simulink model "model_3dof_lateral_carsim"  (R2022a)
settings: Solver=ode5  StartTime=0.0  StopTime=1200  FixedStep=para_sim_step  MaxStep=1e-3  RelTol=1e-3
model workspace (MAT data in the model file):
  SCD_FRESTIMATE_Operating_Point = opcond.OperatingPoint
  SCD_FRESTIMATE_Operating_Point.Model_ = 'model_1dof_longitudinal'
  SCD_FRESTIMATE_Operating_Point.States_(1) = opcond.StatePoint
  SCD_FRESTIMATE_Operating_Point.States_(1).Nx_ = 41
  SCD_FRESTIMATE_Operating_Point.States_(1).Block_ = 'model_1dof_longitudinal/Excitation System/Int Operator'
  SCD_FRESTIMATE_Operating_Point.States_(1).StateName_ = 'v'
  SCD_FRESTIMATE_Operating_Point.States_(1).x_ = [2.02683501926e-10; 1.37568821264e-19; 7.14890844399e-22; 1.12455204277e-20; -7.0630005675e-20; -6.95938068614e-20; 2.72721447959e-21; -3.93535312325e-20; -1.14815977745e-19; 3.30570889294e-20; 3.78600196645e-20; 7.21851569254e-20; -1.77555585105e-19; -2.35291525241e-20; 4.41713994739e-20; -2.05900764101e-21; -1.58367864176e-20; 6.35039836383e-20; -1.30347120926e-20; 1.28680290784e-21; 5.17371795703e-20; 6.49899736287e-20; -4.65181773693e-21; 5.74556218522e-21; -3.90326541642e-20; -4.95314223748e-20; -4.80167923753e-19; 9.22449192438e-20; -2.20085792962e-21; -4.30092800651e-20; -3.42774380714e-20; -1.20947897418e-20; -3.0642370533e-20; -6.43164282462e-20; -2.97515387843e-19; -1.68698506591e-20; 2.312266433e-19; -7.84373380068e-21; 1.67577252929e-20; 2.59801809162e-21; -7.43993193604e-23]
  SCD_FRESTIMATE_Operating_Point.States_(2) = opcond.StatePoint
  SCD_FRESTIMATE_Operating_Point.States_(2).Nx_ = 1
  SCD_FRESTIMATE_Operating_Point.States_(2).Block_ = 'model_1dof_longitudinal/Vehicle Body 1DOF Longitudinal/Vehicle Body 1 DOF/Bus Creation/Body Frame/Longitudinal 1DOF/Integrator3'
  SCD_FRESTIMATE_Operating_Point.States_(2).x_ = 7.28555022085e-16
  SCD_FRESTIMATE_Operating_Point.States_(3) = opcond.StatePoint
  SCD_FRESTIMATE_Operating_Point.States_(3).Nx_ = 1
  SCD_FRESTIMATE_Operating_Point.States_(3).Block_ = 'model_1dof_longitudinal/Vehicle Body 1DOF Longitudinal/Vehicle Body 1 DOF/Integrator1'
  SCD_FRESTIMATE_Operating_Point.States_(3).x_ = -8.63730588445e-16
  SCD_FRESTIMATE_Operating_Point.States_(4) = opcond.StatePoint
  SCD_FRESTIMATE_Operating_Point.States_(4).Nx_ = 1
  SCD_FRESTIMATE_Operating_Point.States_(4).Block_ = 'model_1dof_longitudinal/Vehicle Body 1DOF Longitudinal/Vehicle Body 1 DOF/Vehicle/Integrator'
  SCD_FRESTIMATE_Operating_Point.States_(4).x_ = 1.82750662194e-20
values from neighbouring files (symbols this model uses):
  para_mats = paraStruct.Sv    [main_lateral.m]    (also in main_steering_lateral.m)
  para_sim_matu = paraStruct.SimUv    [main_lateral.m]    (also in main_steering_lateral.m)
  para_sim_step = 5e-4/2    (= 0.00025)    [main_lateral.m]    (also in main_steering_lateral.m = 0.005)
  para_vinit = paraStruct.VInit    [main_lateral.m]    (also in main_steering_lateral.m)
  sim_iun = Simulink.Parameter(1)    [main_lateral.m]    (also in main_steering_lateral.m)
  sim_usnr = zeros(para_sim_usize, 1)    [main_lateral.m]    (also in main_steering_lateral.m)
  ut_pwr = genPower(sim_ut, para_sim_usize)    [main_lateral.m]    (also in main_steering_lateral.m)
libraries: Solver_SF x1, simulink x1
settings Model: SimulationMode=accelerator  Creator=无垠穹宇  LastModifiedBy=无垠穹宇
settings DataIOCC: SaveOutput=off  SignalLogging=off  DSMLogging=off  SignalLoggingName=yt
settings OptimizationCC: SimCompilerOptimization=on
settings DebuggingCC: AlgebraicLoopMsg=none
settings SFSimCC: SimHardwareAcceleration=native
settings RTWCC: DLArmComputeVersion=19.05

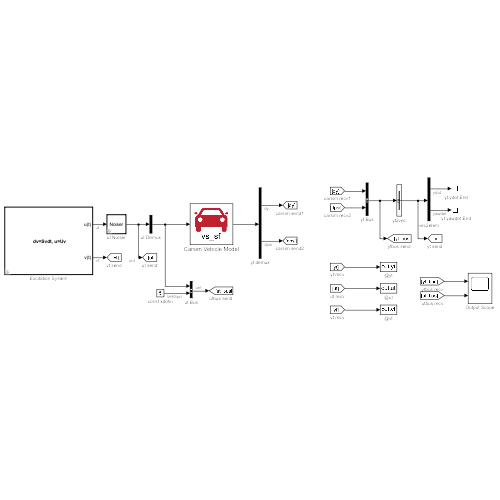
[thumbnail: Simulink's stored preview of the top-level diagram]
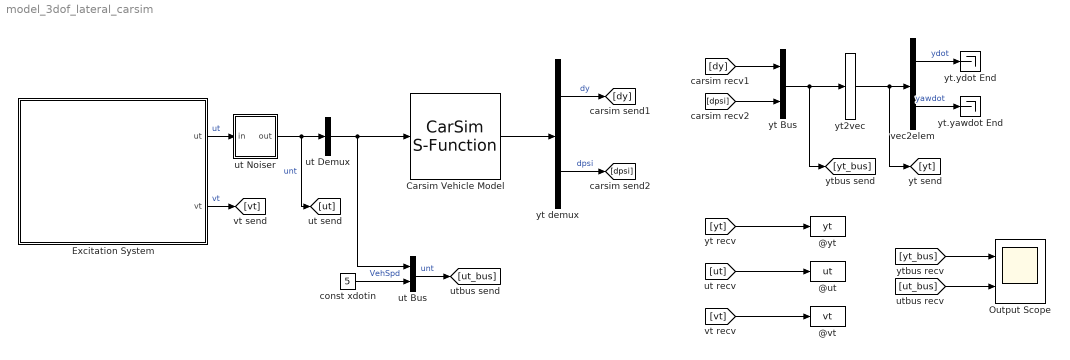
== system model_3dof_lateral_carsim ==
  @ut : ToWorkspace  VariableName=ut  SaveFormat=Timeseries  SampleTime=para_sim_step
      settings: Decimation=para_resamples
  @vt : ToWorkspace  VariableName=vt  SaveFormat=Timeseries  SampleTime=para_sim_step
      settings: Decimation=para_resamples
  @yt : ToWorkspace  VariableName=yt  SaveFormat=Timeseries  SampleTime=para_sim_step
      settings: Decimation=para_resamples
  Carsim Vehicle Model : Solver_SF/CarSim S-Function  Priority=1  SIMFILE=simfile.sim  Run_RTs=off  vs_state_ind=Run  StopMode_ind=Vehicle Model
  Excitation System : Subsystem  TreatAsAtomicUnit=on  mask(State Space with State Vector Output){S=para_mats, U=para_sim_matu, v0=para_vinit}
      mask prompts: S "Matrix S"; U "Matrix U"; v0 "v(0)"
      mask help: 带状态输出的状态空间模型(无控制输入)
      mask DialogControl ParameterGroupVar Prompt: 参数
      mask Display:
      | disp('\bf dv=Svdt, u=Uv', 'texmode', 'on');
      | port_label('output', 1, 'u(t)');
      | port_label('output', 2, 'v(t)');
  Output Scope : Scope  NumInputPorts=2
  const xdotin : Constant  Value=5  VectorParams1D=off  OutDataTypeStr=double
  ut Bus : BusCreator  Inputs=2
  ut Demux : Demux  Outputs=1
  ut Noiser : Subsystem  TreatAsAtomicUnit=on  mask(Vectorized AWGN){pwr=ut_pwr, snr=sim_usnr, tmin=20*para_sim_step, judge_para=sim_iun}
      mask prompts: pwr "信号功率向量 (W)"; snr "信噪比向量   (dB)"; tmin "最小动态时间 (s)"; judge_para "噪声启用判断"
      mask help: 给定信号功率和信噪比, 添加高斯白噪声到信号中
      mask DialogControl ParameterGroupVar Prompt: 参数
      mask Display: disp('Noiser');
  vec2elem : Demux  Outputs=2
  yt Bus : BusCreator  Inputs=2
  yt demux : Demux  Outputs=2
  yt.yawdot End : Terminator
  yt.ydot End : Terminator
  yt2vec : BusToVector
  wires:
  Excitation System/1(ut) -> ut Noiser/1(in)  "ut"
  ut Noiser/1(out) -> ut Demux/1, [ut]  "unt"
  Excitation System/2(vt) -> [vt]  "vt"
  [vt] -> @vt/1
  yt Bus/1 -> yt2vec/1, [yt_bus]
  [ut_bus] -> Output Scope/2
  [ut] -> @ut/1
  [yt_bus] -> Output Scope/1
  [yt] -> @yt/1
  yt2vec/1 -> vec2elem/1, [yt]
  Carsim Vehicle Model/1 -> yt demux/1
  yt demux/1 -> [dy]  "dy"
  yt demux/2 -> [dpsi]  "dpsi"
  const xdotin/1 -> ut Bus/2  "VehSpd"
  ut Bus/1 -> [ut_bus]  "unt"
  ut Demux/1 -> ut Bus/1, Carsim Vehicle Model/1
  [dy] -> yt Bus/1
  [dpsi] -> yt Bus/2
  vec2elem/1 -> yt.ydot End/1  "ydot"
  vec2elem/2 -> yt.yawdot End/1  "yawdot"

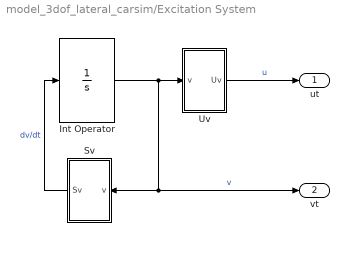
== system model_3dof_lateral_carsim/Excitation System ==
  Int Operator : Integrator  InitialCondition=v0  ContinuousStateAttributes='v'
  Sv : Subsystem
      mask Display: disp('Sv');
  Uv : Subsystem
      mask Display: disp('Uv');
  ut : Outport  OutDataTypeStr=double
  vt : Outport  Port=2  OutDataTypeStr=double
  wires:
  Uv/1(Uv) -> ut/1  "u"
  Int Operator/1 -> Uv/1(v), vt/1, Sv/1(v)  "v"
  Sv/1(Sv) -> Int Operator/1  "dv/dt"

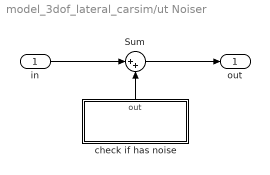
== system model_3dof_lateral_carsim/ut Noiser ==
  in : Inport  OutDataTypeStr=double
  Sum : Sum  Inputs=|++  AccumDataTypeStr=double  OutDataTypeStr=double
  check if has noise : Subsystem  Variant=on
      mask Display: disp('Variant: awgn/zeros');
  out : Outport  OutDataTypeStr=double
  wires:
  in/1 -> Sum/1
  Sum/1 -> out/1
  check if has noise/1(out) -> Sum/2

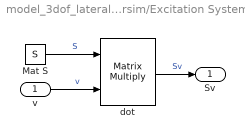
== system model_3dof_lateral_carsim/Excitation System/Sv ==
  v : Inport  OutDataTypeStr=double
  Mat S : Constant  Value=S  VectorParams1D=off  OutDataTypeStr=double
  dot : Product  Multiplication=Matrix(*)  InputSameDT=on  OutDataTypeStr=double
  Sv : Outport  OutDataTypeStr=double
  wires:
  dot/1 -> Sv/1  "Sv"
  v/1 -> dot/2  "v"
  Mat S/1 -> dot/1  "S"

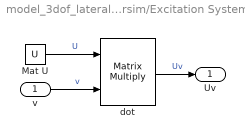
== system model_3dof_lateral_carsim/Excitation System/Uv ==
  v : Inport  OutDataTypeStr=double
  Mat U : Constant  Value=U  VectorParams1D=off  OutDataTypeStr=double
  dot : Product  Multiplication=Matrix(*)  InputSameDT=on  OutDataTypeStr=double
  Uv : Outport  OutDataTypeStr=double
  wires:
  dot/1 -> Uv/1  "Uv"
  Mat U/1 -> dot/1  "U"
  v/1 -> dot/2  "v"

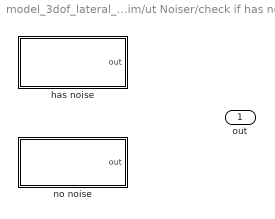
== system model_3dof_lateral_carsim/ut Noiser/check if has noise ==
  has noise : Subsystem  TreatAsAtomicUnit=on  VariantControl=judge_para == 0
  no noise : Subsystem  TreatAsAtomicUnit=on  VariantControl=judge_para ~= 0
  out : Outport  OutDataTypeStr=double

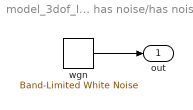
== system model_3dof_lateral_carsim/ut Noiser/check if has noise/has noise ==
  wgn : simulink/Sources/Band-Limited White Noise  Cov=pwr./(10.^(snr./10)).*(2*pi*tmin/100)  Ts=(1/20)*tmin  seed=[23341]
  out : Outport  OutDataTypeStr=double
  wires:
  wgn/1 -> out/1

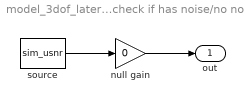
== system model_3dof_lateral_carsim/ut Noiser/check if has noise/no noise ==
  null gain : Gain  Gain=0  ParamDataTypeStr=double  OutDataTypeStr=double
  source : Constant  Value=sim_usnr  OutDataTypeStr=double
  out : Outport
  wires:
  null gain/1 -> out/1
  source/1 -> null gain/1
